simulink model "encrypted_teleoperation_2021a"  (R2022a)
settings: Solver=ode5  StartTime=0.0  StopTime=10  FixedStep=0.001  MaxStep=Ts  RelTol=1e-3
model workspace (MAT data in the model file):
  Ts = 0.02
  benv = Simulink.Parameter
  benv.Value = 13.5
  benv.DataType = 'auto'
  benv.Complexity = 'real'
  benv.Dimensions = [1 1]
  bm = Simulink.Parameter
  bm.Value = 0.1
  bm.DataType = 'auto'
  bm.Complexity = 'real'
  bm.Dimensions = [1 1]
  bms = Simulink.Parameter
  bms.Value = 23.5
  bms.DataType = 'auto'
  bms.Complexity = 'real'
  bms.Dimensions = [1 1]
  bs = Simulink.Parameter
  bs.Value = 0.1
  bs.DataType = 'auto'
  bs.Complexity = 'real'
  bs.Dimensions = [1 1]
  ctrl_slct = Simulink.Parameter
  ctrl_slct.Value = 1
  ctrl_slct.DataType = 'auto'
  ctrl_slct.Complexity = 'real'
  ctrl_slct.Dimensions = [1 1]
  fm = Simulink.Parameter
  fm.Value = 1
  fm.DataType = 'auto'
  fm.Complexity = 'real'
  fm.Dimensions = [1 1]
  kenv = Simulink.Parameter
  kenv.Value = 50
  kenv.DataType = 'auto'
  kenv.Complexity = 'real'
  kenv.Dimensions = [1 1]
  kms = Simulink.Parameter
  kms.Value = 150
  kms.DataType = 'auto'
  kms.Complexity = 'real'
  kms.Dimensions = [1 1]
  mm = Simulink.Parameter
  mm.Value = 1
  mm.DataType = 'auto'
  mm.Complexity = 'real'
  mm.Dimensions = [1 1]
  mms = Simulink.Parameter
  mms.Value = 0.5
  mms.DataType = 'auto'
  mms.Complexity = 'real'
  mms.Dimensions = [1 1]
  ms = Simulink.Parameter
  ms.Value = 1
  ms.DataType = 'auto'
  ms.Complexity = 'real'
  ms.Dimensions = [1 1]
  um = Simulink.Parameter
  um.Value = 0.1
  um.DataType = 'auto'
  um.Complexity = 'real'
  um.Dimensions = [1 1]
  us = Simulink.Parameter
  us.Value = 0.1
  us.DataType = 'auto'
  us.Complexity = 'real'
  us.Dimensions = [1 1]
  xbar = Simulink.Parameter
  xbar.Value = 0.1
  xbar.DataType = 'auto'
  xbar.Complexity = 'real'
  xbar.Dimensions = [1 1]
libraries: simulink x6
settings Model: PauseTimes=1.3  Creator=jueda3  LastModifiedBy=xzhao
settings SolverCC: AlgebraicLoopSolver=TrustRegion  AutoInsertRateTranBlk=on
settings DataIOCC: LimitDataPoints=on  SaveFormat=Array  SignalLoggingSaveFormat=ModelDataLogs  ReturnWorkspaceOutputs=off  SignalLoggingName=sigsOut
settings OptimizationCC: DefaultParameterBehavior=Inlined  EnhancedBackFolding=on  PassReuseOutputArgsAs=Individual arguments  ZeroExternalMemoryAtStartup=off  ZeroInternalMemoryAtStartup=off  OptimizeBlockOrder=speed  DifferentSizesBufferReuse=on  OptimizationCustomize=off  EfficientTunableParamExpr=on
settings DebuggingCC: SaveWithParameterizedLinksMsg=none  UnderspecifiedInitializationDetection=Classic  MergeDetectMultiDrivingBlocksExec=none  SignalResolutionControl=TryResolveAllWithWarning  MultiTaskDSMMsg=warning  MultiTaskCondExecSysMsg=none  ParameterTunabilityLossMsg=error  UnconnectedInputMsg=warning  UnconnectedOutputMsg=warning  UnconnectedLineMsg=warning  SFMachineParentedDataDiag=warning  ArithmeticOperatorsInVariantConditions=warning
settings HardwareCC: ProdBitPerPointer=32  ProdBitPerSizeT=32  ProdBitPerPtrDiffT=32  ProdLargestAtomicFloat=None  ProdIntDivRoundTo=Undefined  ProdEndianess=Unspecified  ProdWordSize=32  ProdHWDeviceType=32-bit Generic  TargetBitPerPointer=64  TargetBitPerSizeT=64  TargetBitPerPtrDiffT=64  TargetLongLongMode=on  TargetIntDivRoundTo=Zero  TargetEndianess=LittleEndian  TargetWordSize=64  TargetHWDeviceType=MATLAB Host  ProdEqTarget=off
settings ModelReferenceCC: PropagateSignalLabelsOutOfModel=off
settings SFSimCC: SimUseLocalCustomCode=off  MATLABDynamicMemAlloc=off  CustomCodeUndefinedFunction=UseInterfaceOnly
settings RTWCC: Description=Embedded Coder (host-based shared library target)  SystemTargetFile=ert_shrlib.tlc  TemplateMakefile=ert_default_tmf  RTWUseLocalCustomCode=off  DLArmComputeVersion=19.05
settings CodeAppCC: ForceParamTrailComments=on  IgnoreCustomStorageClasses=off  OperatorAnnotations=on  SimulinkDataObjDesc=on  SFDataObjDesc=on  InsertBlockDesc=on
settings STFCustomTargetCC: MultiwordLength=256  GenerateSampleERTMain=on  ParMdlRefBuildCompliant=on  CompOptLevelCompliant=on  CombineOutputUpdateFcns=on  ERTCustomFileBanners=on  SupportContinuousTime=off  SupportNonInlinedSFcns=off  RemoveResetFunc=on  MATLABClassNameForMDSCustomization=Simulink.SoftwareTarget.ERTCustomization  ModelStepFunctionPrototypeControlCompliant=on  GRTInterface=off  UseToolchainInfoCompliant=on  SystemTargetFile=ert_shrlib.tlc
settings ERTTargetCC: GenerateSampleERTMain=on  ConcurrentExecutionCompliant=off  CPPClassGenCompliant=off  InlinedParameterPlacement=NonHierarchical  ERTCustomFileTemplate=example_file_process.tlc
settings ConfigComp: CovMetricSettings=dw  CovSaveCumulativeToWorkspaceVar=on  CovSaveSingleToWorkspaceVar=on  CovExternalEMLEnable=off

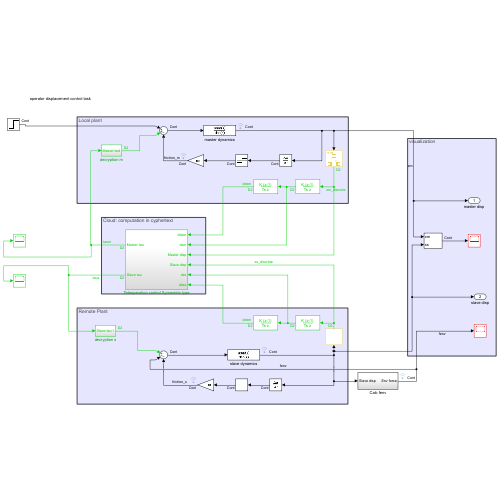
[thumbnail: Simulink's stored preview of the top-level diagram]
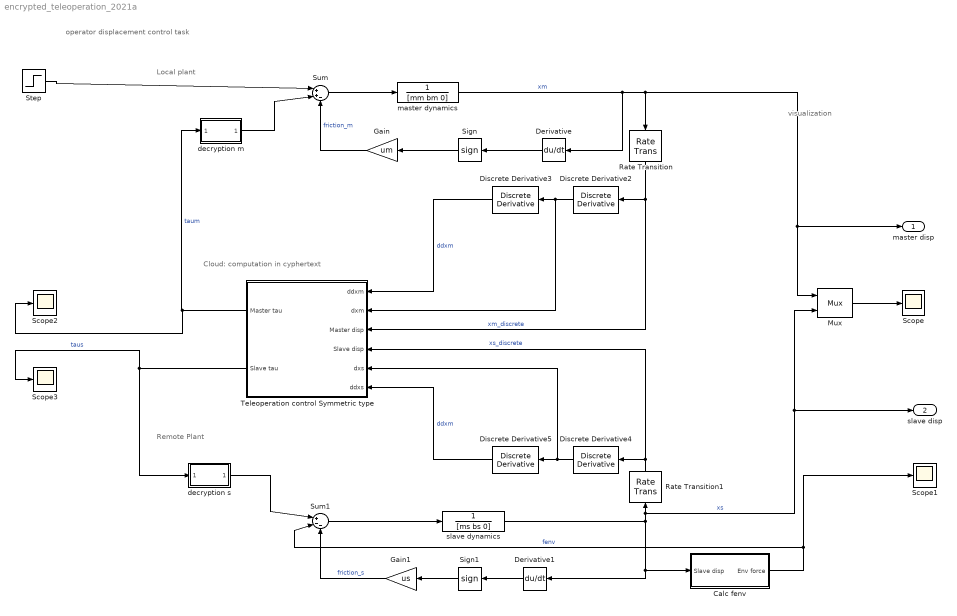
== system encrypted_teleoperation_2021a ==
  note: visualization
  note: Remote Plant
  note: Local plant
  note: Cloud: computation in cyphertext
  note: operator displacement control task
  Calc fenv : Subsystem
  Derivative : Derivative  CoefficientInTFapproximation=0.01
  Derivative1 : Derivative  CoefficientInTFapproximation=0.01
  Discrete Derivative{2..5} (4 alike) : simulink/Discrete/Discrete Derivative  gainval=1.0  ICPrevScaledInput=0.0  OutMin=[]  OutMax=[]  OutDataType=fixdt(1, 16)  OutScaling=2^-10  DoSatur=off
  Gain : Gain  Gain=um
  Gain1 : Gain  Gain=us
  Mux : Mux  Inputs=2
      settings: DisplayOption=signals
  Rate Transition : RateTransition  OutPortSampleTime=Ts
  Rate Transition1 : RateTransition  OutPortSampleTime=Ts
  Scope{,1..3} (4 alike) : Scope
  Sign : Signum
  Sign1 : Signum
  Step : Step  After=fm  SampleTime=0
  Sum : Sum  Inputs=|++-
  Sum1 : Sum  Inputs=|+--
  Teleoperation control Symmetric type : Subsystem
  decryption m : Subsystem
  decryption s : Subsystem
  master dynamics : TransferFcn  Denominator=[mm bm 0]
  slave dynamics : TransferFcn  Denominator=[ms bs 0]
  master disp : Outport
  slave disp : Outport  Port=2
  wires:
  slave dynamics/1 -> Rate Transition1/1, slave disp/1, Mux/2, Calc fenv/1(Slave disp), Derivative1/1  "xs"
  Mux/1 -> Scope/1
  Teleoperation control Symmetric type/2(Slave tau) -> Scope3/1, decryption s/1(Slave tau)  "taus"
  Teleoperation control Symmetric type/1(Master tau) -> Scope2/1, decryption m/1(Master tau)  "taum"
  Sum/1 -> master dynamics/1
  master dynamics/1 -> master disp/1, Mux/1, Rate Transition/1, Derivative/1  "xm"
  Calc fenv/1(Env force) -> Scope1/1, Sum1/2  "fenv"
  Gain/1 -> Sum/3  "friction_m"
  Sum1/1 -> slave dynamics/1
  Gain1/1 -> Sum1/3  "friction_s"
  Sign1/1 -> Gain1/1
  Rate Transition/1 -> Teleoperation control Symmetric type/3(Master disp), Discrete Derivative2/1  "xm_discrete"
  Rate Transition1/1 -> Teleoperation control Symmetric type/4(Slave disp), Discrete Derivative4/1  "xs_discrete"
  decryption m/1(Out1) -> Sum/2
  decryption s/1(Out1) -> Sum1/1
  Step/1 -> Sum/1
  Discrete Derivative2/1 -> Discrete Derivative3/1, Teleoperation control Symmetric type/2(dxm)
  Discrete Derivative3/1 -> Teleoperation control Symmetric type/1(ddxm)  "ddxm"
  Discrete Derivative4/1 -> Teleoperation control Symmetric type/5(dxs), Discrete Derivative5/1
  Discrete Derivative5/1 -> Teleoperation control Symmetric type/6(ddxs)  "ddxm"
  Sign/1 -> Gain/1
  Derivative/1 -> Sign/1
  Derivative1/1 -> Sign1/1

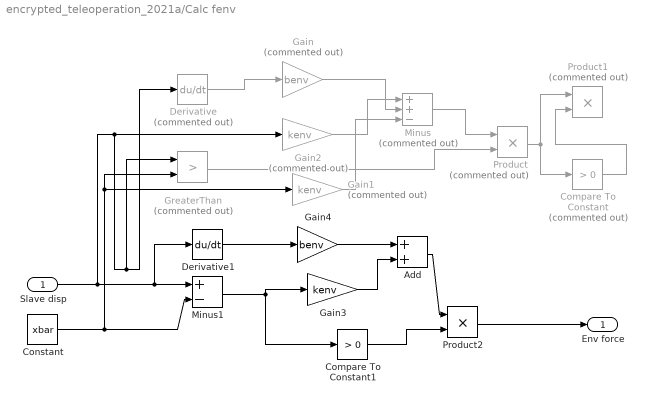
== system encrypted_teleoperation_2021a/Calc fenv ==
  Slave disp : Inport
  Add : Sum
  Compare To Constant : simulink/Logic and Bit Operations/Compare To Constant  Commented=on  relop=>  const=0  OutDataTypeStr=boolean
  Compare To Constant1 : simulink/Logic and Bit Operations/Compare To Constant  relop=>  const=0  OutDataTypeStr=boolean
  Constant : Constant  Value=xbar
  Derivative : Derivative  Commented=on
  Derivative1 : Derivative
  Gain : Gain  Commented=on  Gain=benv
  Gain1 : Gain  Commented=on  Gain=kenv
  Gain2 : Gain  Commented=on  Gain=kenv
  Gain3 : Gain  Gain=kenv
  Gain4 : Gain  Gain=benv
  GreaterThan : RelationalOperator  Commented=on  Operator=>  OutDataTypeStr=boolean  RndMeth=Simplest  InputSameDT=off
  Minus : Sum  Commented=on  Inputs=++-
  Minus1 : Sum  Inputs=+-
  Product : Product  Commented=on
  Product1 : Product  Commented=on
  Product2 : Product
  Env force : Outport
  wires:
  Slave disp/1 -> Gain2/1, Derivative/1, GreaterThan/1, Derivative1/1, Minus1/1
  Gain2/1 -> Minus/1
  Product/1 -> Compare To Constant/1, Product1/1
  Constant/1 -> GreaterThan/2, Gain1/1, Minus1/2
  GreaterThan/1 -> Product/2
  Gain1/1 -> Minus/3
  Minus/1 -> Product/1
  Derivative/1 -> Gain/1
  Gain/1 -> Minus/2
  Compare To Constant/1 -> Product1/2
  Minus1/1 -> Compare To Constant1/1, Gain3/1
  Gain3/1 -> Add/2
  Compare To Constant1/1 -> Product2/2
  Product2/1 -> Env force/1
  Derivative1/1 -> Gain4/1
  Gain4/1 -> Add/1
  Add/1 -> Product2/1

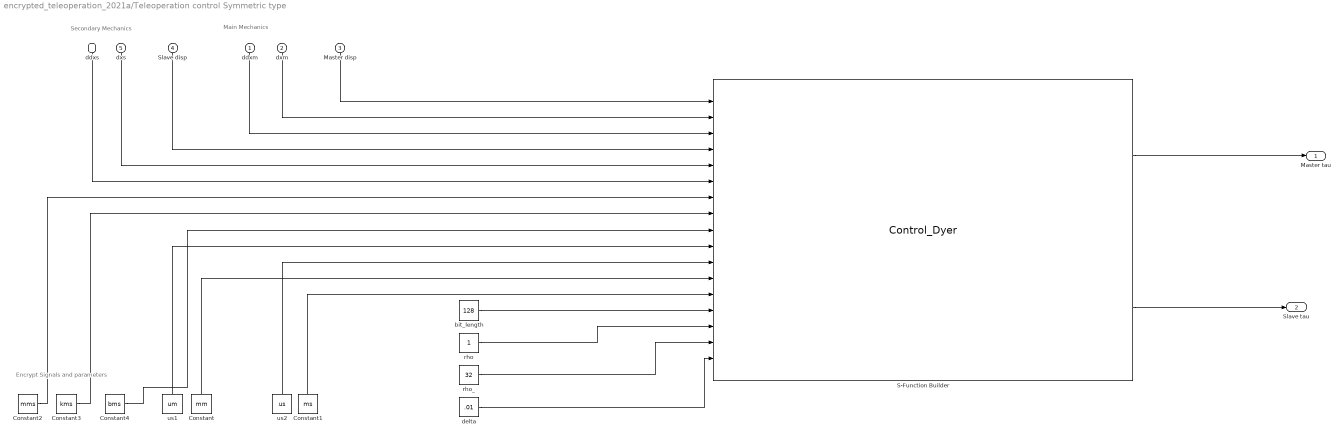
== system encrypted_teleoperation_2021a/Teleoperation control Symmetric type ==
  note: Encrypt Signals and parameters
  note: Secondary Mechanics
  note: Main Mechanics
  ddxm : Inport
  dxm : Inport  Port=2
  Master disp : Inport  Port=3
  Slave disp : Inport  Port=4
  dxs : Inport  Port=5
  ddxs : Inport  Port=6
  Constant : Constant  Value=mm
  Constant1 : Constant  Value=ms
  Constant2 : Constant  Value=mms
  Constant3 : Constant  Value=kms
  Constant4 : Constant  Value=bms
  S-Function Builder : S-Function  FunctionName=Control_Dyer  Parameters=1  SFunctionModules=Control_Dyer_wrapper  SFunctionDeploymentMode=off  EnableBusSupport=off  mask(S-Function Builder){}
      mask help: Simulink:masks:SFunctionBuilder_MD
      mask init:
      | val = [[.9  0.75 0.75 1 1 .9 .9 1]',[1 1 0.75 0.75 .9 .9 1 .9]'];try , sys = get_param(gcb,'SfunBuilderFcnName');if isempty(sys), sys = get_param(gcb,'FunctionName'); end,catch, sys = get_param(gcb,'FunctionName'); end
      settings: CopyFcn=set_param(gcbh,'LinkStatus','none')  OpenFcn=sfunctionwizard(gcbh)
      mask Display:
      | plot(val(:,1),val(:,2))
      | disp(sys)
      | port_label('input',1,'xm')
      | port_label('input',2,'dxm')
      | port_label('input',3,'ddxm')
      | port_label('input',4,'xs')
      | port_label('input',5,'dxs')
      | port_label('input',6,'ddxs')
      | port_label('input',7,'mms')
      | port_label('input',8,'kms')
      | port_label('input',9,'bms')
      | port_label('input',10,'um')
      | port_label('input',11,'us')
      | port_label('input',12,'mm')
      | port_label('input',13,'ms')
      | port_label('input',14,'bit_length')
      | port_label('input',15,'rho')
      | port_label('input',16,'rho_')
      | port_label('input',17,'delta')
      | port_label('output',1,'tau_m')
      | port_label('output',2,'tau_s')
  bit_length : Constant  Value=128
  delta : Constant  Value=.01
  rho : Constant
  rho_ : Constant  Value=32
  us1 : Constant  Value=um
  us2 : Constant  Value=us
  Master tau : Outport
  Slave tau : Outport  Port=2
  wires:
  Master disp/1 -> S-Function Builder/1
  Slave disp/1 -> S-Function Builder/4
  Constant2/1 -> S-Function Builder/7
  Constant3/1 -> S-Function Builder/8
  Constant4/1 -> S-Function Builder/9
  us1/1 -> S-Function Builder/10
  us2/1 -> S-Function Builder/11
  Constant/1 -> S-Function Builder/12
  Constant1/1 -> S-Function Builder/13
  dxm/1 -> S-Function Builder/2
  ddxm/1 -> S-Function Builder/3
  dxs/1 -> S-Function Builder/5
  ddxs/1 -> S-Function Builder/6
  S-Function Builder/1 -> Master tau/1
  S-Function Builder/2 -> Slave tau/1
  bit_length/1 -> S-Function Builder/14
  rho/1 -> S-Function Builder/15
  rho_/1 -> S-Function Builder/16
  delta/1 -> S-Function Builder/17

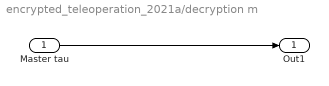
== system encrypted_teleoperation_2021a/decryption m ==
  Master tau : Inport
  Out1 : Outport
  wires:
  Master tau/1 -> Out1/1

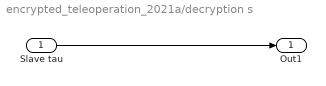
== system encrypted_teleoperation_2021a/decryption s ==
  Slave tau : Inport
  Out1 : Outport
  wires:
  Slave tau/1 -> Out1/1
